simulink model "buoyancy_simulation"  (R2025a)
settings: Solver=VariableStepAuto  StartTime=0.0  StopTime=100  FixedStep=0.01  RelTol=1e-3
InitFcn:
  | parameters
values from neighbouring files (symbols this model uses):
  A = pi*(d/2)^2    (= 0.00785398163397)    [parameters.m]    (also in simulations_code.m; test.m)
  A_cross = 0.07    [parameters.m]    (also in simulations_code.m; test.m)
  C_d = 1.0    (= 1)    [parameters.m]    (also in simulations_code.m; test.m)
  F_pos = 2.94 + m*g    (= 32.37)    [parameters.m]    (also in sensitivity.m = 0.300 * g + m_values(i)*g; simulation_matlab.m = 2.94; simulations_code.m; test.m)
  g = 9.81    [parameters.m]    (also in simulation_matlab.m; simulations_code.m; test.m)
  k_m = 50    [parameters.m]    (also in simulation_matlab.m; simulations_code.m = 5; test.m = 5)
  m = 3    [parameters.m]    (also in simulation_matlab.m; simulations_code.m; test.m)
  m_a = 2.5    [parameters.m]    (also in simulation_matlab.m = 0; simulations_code.m; test.m)
  p = 0.002    [parameters.m]    (also in simulation_matlab.m; simulations_code.m; test.m)
  rho = 1000    [parameters.m]    (also in simulation_matlab.m; simulations_code.m; test.m)
libraries: slpidlib x1
settings Model: Creator=hannasennero  LastModifiedBy=hannasennero
settings SolverCC: ZeroCrossAlgorithm=Adaptive
settings DebuggingCC: IgnoredZcDiagnostic=none

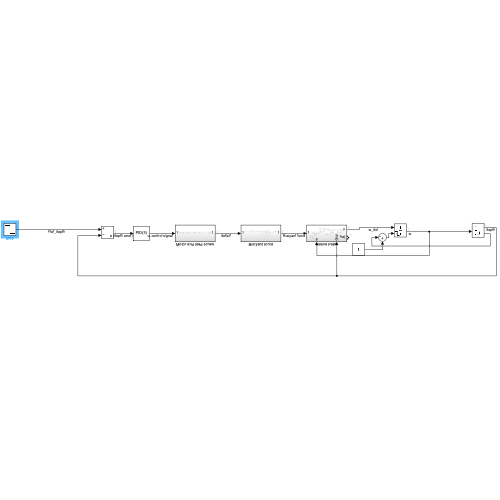
[thumbnail: Simulink's stored preview of the top-level diagram]
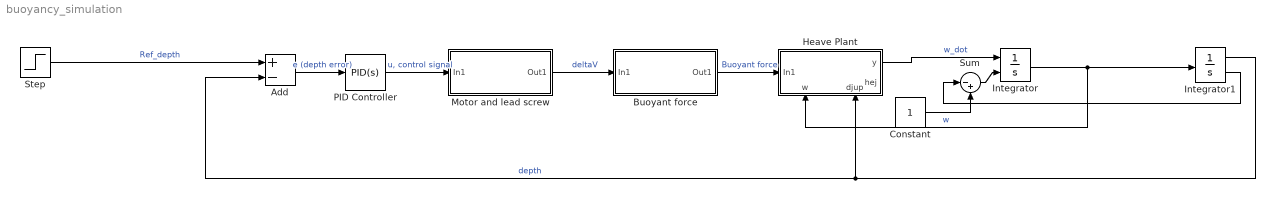
== system buoyancy_simulation ==
  Add : Sum  Inputs=+-
  Buoyant force : Subsystem
  Constant : Constant
  Heave Plant : Subsystem
      settings: PortSchema="{\"entries\":[{\"content\":{\"sides\":[{\"content\":{\"connectorIds\":[\"In1\"]},\"type\":\"ConnectorPlacement.EquallySpacedRectSide\",\"uuid\":\"64163796-67b4-4874-a81c-abb8813ac274\"},{\"content\":{\"connectorIds\":[\"Out1\",\"Out2\"],\"side\":\"RIGHT\"},\"type\":\"ConnectorPlacement.EquallySpacedRectSide\",\"uuid\":\"c10edb53-fdb3-4b5f-a96a-74da846fe7c3\"},{\"content\":{\"side\":\"TOP\"},\"type\":\"ConnectorPlacement.EquallySpacedRectSide\",\"uuid\":\"03a8d6bf-bc70-4644-992b-47d9b15e439c\"},{\"content\":{\"connectorIds\":[\"In2\",\"In3\"],\"side\":\"BOTTOM\"},\"type\":\"ConnectorPlacement.EquallySpacedRectSide\",\"uuid\":\"3bbf4b5d-45ae-4ac2-bdf5-5e5dee5a19eb\"}]},\"type\":\"ConnectorPlacement.EquallySpacedConnector\",\"uuid\":\"f3efd6ea-c772-4fc4-945d-e21c2b4b2ad1\"}],\"packageUris\":[\"http://schema.mathworks.com/mf0/Connector/R2020b\"],\"version\":\"1.0\"}"
  Integrator : Integrator  ExternalReset=falling  ZeroCross=off
  Integrator1 : Integrator  LimitOutput=on  LowerSaturationLimit=0  ShowSaturationPort=on
  Motor and lead screw : Subsystem
  PID Controller : slpidlib/PID Controller  Controller=PID  Form=Parallel  TimeDomain=Continuous-time  UseExternalTs=off  SampleTime=-1  IntegratorMethod=Forward Euler  FilterMethod=Forward Euler  ControllerParametersSource=internal  P=10  I=0.1  UseKiTs=off  D=20  UseExternalDerivativeSource=off  N=0  UseFilter=on  TunerSelectOption=Transfer Function Based (PID Tuner App)  InitialConditionSource=internal  InitialConditionForIntegrator=0  InitialConditionForFilter=0  DifferentiatorICPrevScaledInput=0  ExternalReset=none  TrackingMode=off  Kt=1  LimitOutput=off  SatLimitsSource=internal  UpperSaturationLimit=inf  LowerSaturationLimit=-inf  LinearizeAsGain=on  AntiWindupMode=none  Kb=1  LimitIntegrator=off  UpperIntegratorSaturationLimit=inf  LowerIntegratorSaturationLimit=-inf  POutMin=[]  POutMax=[]  IOutMin=[]  IOutMax=[]  DOutMin=[]  DOutMax=[]  NOutMin=[]  NOutMax=[]  SumOutMin=[]  SumOutMax=[]  SaturationOutMin=[]  SaturationOutMax=[]  PParamMin=[]  PParamMax=[]  IParamMin=[]  IParamMax=[]  DParamMin=[]  DParamMax=[]  NParamMin=[]  NParamMax=[]  KbParamMin=[]  KbParamMax=[]  KtParamMin=[]  KtParamMax=[]  KbOutMin=[]  KbOutMax=[]  KtOutMin=[]  KtOutMax=[]  IntegratorOutMin=[]  IntegratorOutMax=[]  FilterOutMin=[]  FilterOutMax=[]  SumI1OutMin=[]  SumI1OutMax=[]  SumI2OutMin=[]  SumI2OutMax=[]  SumI3OutMin=[]  SumI3OutMax=[]  SumI4OutMin=[]  SumI4OutMax=[]  SumDOutMin=[]  SumDOutMax=[]  DifferentiatorOutMin=[]  DifferentiatorOutMax=[]  FilterDiffOutCoefMin=[]  FilterDiffOutCoefMax=[]  ReciprocalOutMin=[]  ReciprocalOutMax=[]  SumDenOutMin=[]  SumDenOutMax=[]  SumNumOutMin=[]  SumNumOutMax=[]  DivideOutMin=[]  DivideOutMax=[]  UdiffTsProdOutMin=[]  UdiffTsProdOutMax=[]  NTsProdOutMin=[]  NTsProdOutMax=[]  UintegralTsProdOutMin=[]  UintegralTsProdOutMax=[]  UngainTsProdOutMin=[]  UngainTsProdOutMax=[]  ClampingZeroOutDataTypeStr=Inherit: Inherit via back propagation  ClampingZeroOutMin=[]  ClampingZeroOutMax=[]  FilterDenConstantOutDataTypeStr=Inherit: Inherit via back propagation  FilterDenConstantOutMin=[]  FilterDenConstantOutMax=[]  PCopyOutDataTypeStr=Inherit: Inherit via back propagation  PCopyOutMin=[]  PCopyOutMax=[]  NCopyOutDataTypeStr=Inherit: Inherit via back propagation  NCopyOutMin=[]  NCopyOutMax=[]  IntegratorContinuousStateAttributes=''  IntegratorStateMustResolveToSignalObject=off  IntegratorRTWStateStorageClass=Auto  FilterContinuousStateAttributes=''  FilterStateMustResolveToSignalObject=off  FilterRTWStateStorageClass=Auto  ParallelPVariant=InternalParameters  IdealPVariant=Disabled  IVariant=InternalParameters  DVariant=InternalParameters  IntegratorVariant=Continuous  SatVariant=Disabled  AWVariant=Passthrough  PCopyVariant=Disabled  TRVariant=Disabled  FdbkBlocksVariant=Forward  IdealPFdbkVariant=Disabled  SatFdbkVariant=Disabled  DerivativeFilterVariant=ContFilter  NVariant=InternalParameters  NCopyVariant=Disabled  FilterICVariant=InternalICsFilter  IntegratorICVariant=InternalICs  ExternalResetVariant=Disabled  TRSumVariant=Passthrough  SumFdbkVariant=Disabled  SumVariant=Sum_PID  TsampFilterVariant=InternalTs  TsampNgainVariant=Passthrough  TsampIntegralVariant=Disabled_SignalSpec  ExternalSaturationOutDataTypeStr=Inherit: Same as second input  DerivativeSourceVariant=ErrorSignal  PreIntVariant=InternalPreInt
  Step : Step  After=-3  SampleTime=0
  Sum : Sum  Inputs=|-+
  wires:
  Step/1 -> Add/1  "Ref_depth"
  Heave Plant/1(y) -> Integrator/1  "w_dot"
  Add/1 -> PID Controller/1  "e (depth error)"
  PID Controller/1 -> Motor and lead screw/1(In1)  "u, control signal"
  Motor and lead screw/1(Out1) -> Buoyant force/1(In1)  "deltaV"
  Buoyant force/1(Out1) -> Heave Plant/1(In1)  "Buoyant force"
  Integrator/1 -> Integrator1/1, Heave Plant/2(w)  "w"
  Integrator1/1 -> Add/2, Heave Plant/3(djup)  "depth"
  Constant/1 -> Sum/2
  Sum/1 -> Integrator/2
  Integrator1/2 -> Sum/1

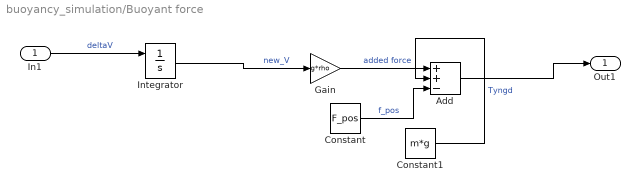
== system buoyancy_simulation/Buoyant force ==
  In1 : Inport
  Add : Sum  Inputs=++-
  Constant : Constant  Value=F_pos
  Constant1 : Constant  Value=m*g
  Gain : Gain  Gain=g*rho
  Integrator : Integrator  ExternalReset=falling  LimitOutput=on  UpperSaturationLimit=0.0005  LowerSaturationLimit=0
  Out1 : Outport
  wires:
  In1/1 -> Integrator/1  "deltaV"
  Add/1 -> Out1/1
  Gain/1 -> Add/1  "added force"
  Constant/1 -> Add/3  "f_pos"
  Constant1/1 -> Add/2  "Tyngd"
  Integrator/1 -> Gain/1  "new_V"

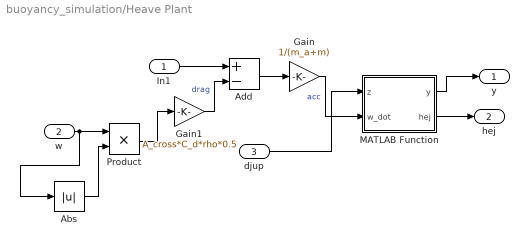
== system buoyancy_simulation/Heave Plant ==
  In1 : Inport
  w : Inport  Port=2
  djup : Inport  Port=3
  Abs : Abs  SaturateOnIntegerOverflow=off
  Add : Sum  Inputs=+-
  Gain : Gain  Gain=1/(m_a+m)
  Gain1 : Gain  Gain=A_cross*C_d*rho*0.5
  MATLAB Function : MATLAB Function  TreatAsAtomicUnit=on
  Product : Product
  y : Outport
  hej : Outport  Port=2
  wires:
  Add/1 -> Gain/1
  Gain1/1 -> Add/2  "drag"
  In1/1 -> Add/1
  MATLAB Function/1(y) -> y/1
  djup/1 -> MATLAB Function/1(z)
  Gain/1 -> MATLAB Function/2(w_dot)  "acc"
  MATLAB Function/2(hej) -> hej/1
  w/1 -> Product/1, Abs/1
  Abs/1 -> Product/2
  Product/1 -> Gain1/1

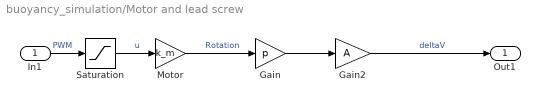
== system buoyancy_simulation/Motor and lead screw ==
  In1 : Inport
  Gain : Gain  Gain=p
  Gain2 : Gain  Gain=A
  Motor : Gain  Gain=k_m
  Saturation : Saturate  UpperLimit=1e-4/k_m/p/A  LowerLimit=-1e-4/k_m/p/A
  Out1 : Outport
  wires:
  Motor/1 -> Gain/1  "Rotation"
  Gain/1 -> Gain2/1
  Gain2/1 -> Out1/1  "deltaV"
  In1/1 -> Saturation/1  "PWM"
  Saturation/1 -> Motor/1  "u"

== matlab function buoyancy_simulation/Heave Plant/MATLAB Function ==
  data: z input; y output; w_dot input; hej output
function [y, hej]= fcn(z,w_dot)
    if z <= 0 && w_dot < 0
        y = 0;
        hej = 20;
    else 
        y = w_dot;
        hej = 0;
    end
